simulink model "rot3"  (R2015b)
settings: Solver=ode45  StartTime=0.0  StopTime=10.0  RelTol=1e-3
settings Model: Creator=sebastian  LastModifiedBy=aleram
settings DataIOCC: SaveFormat=Array
settings DebuggingCC: SolverPrmCheckMsg=warning
settings HardwareCC: ProdBitPerPointer=32  ProdLargestAtomicFloat=None  ProdIntDivRoundTo=Undefined  ProdEndianess=Unspecified  ProdWordSize=32  ProdHWDeviceType=32-bit Generic
settings GRTTargetCC: GeneratePreprocessorConditionals=Disable all
settings ConfigComp: CovModelRefEnable=Off  CovSFcnEnable=off

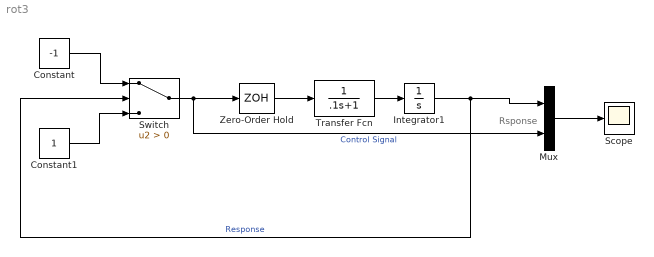
== system rot3 ==
  note: Rsponse
  Constant : Constant  Value=-1
  Constant1 : Constant
  Integrator1 : Integrator  InitialCondition=1
  Mux : Mux  Inputs=2
  Scope : Scope
  Switch : Switch  Criteria=u2 > Threshold
  Transfer Fcn : TransferFcn  Denominator=[.1 1]
  Zero-Order Hold : ZeroOrderHold  SampleTime=0.01
  wires:
  Constant/1 -> Switch/1
  Constant1/1 -> Switch/3
  Mux/1 -> Scope/1
  Integrator1/1 -> Mux/1, Switch/2  "Response"
  Switch/1 -> Zero-Order Hold/1, Mux/2  "Control Signal"
  Transfer Fcn/1 -> Integrator1/1
  Zero-Order Hold/1 -> Transfer Fcn/1
